simulink model "robot_etu"  (R2022a)
settings: Solver=VariableStepAuto  StartTime=0.0  StopTime=10  RelTol=1e-3
values from neighbouring files (symbols this model uses):
  K = -place(A,B,V)    [matrices.m]
undefined symbols (not defined in the file or in its folder): DiscIntNeverNeededParam, ue, x0, xe
libraries: simulink x1
settings Model: Creator=acanon  LastModifiedBy=acanon

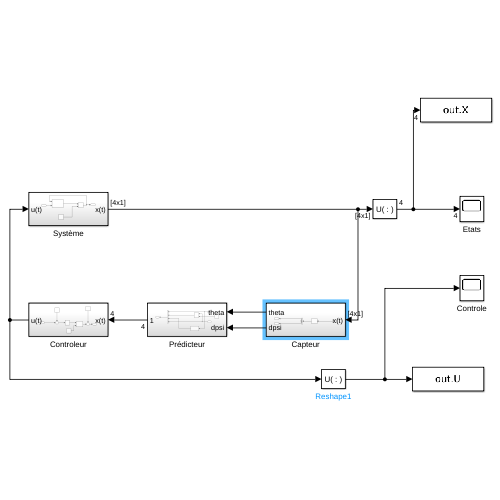
[thumbnail: Simulink's stored preview of the top-level diagram]
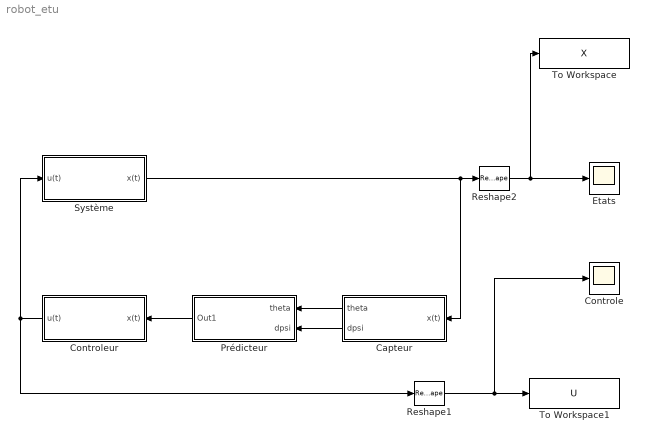
== system robot_etu ==
  Capteur : Subsystem
  Controle : Scope
  Controleur : Subsystem
  Etats : Scope
  Prédicteur : Subsystem
  Reshape1 : Reshape
  Reshape2 : Reshape
  Système : Subsystem
  To Workspace : ToWorkspace  VariableName=X  SaveFormat=Timeseries  SampleTime=-1
  To Workspace1 : ToWorkspace  VariableName=U  SaveFormat=Timeseries  SampleTime=-1
  wires:
  Controleur/1(u(t)) -> Système/1(u(t)), Reshape1/1
  Prédicteur/1(Out1) -> Controleur/1(x(t))
  Capteur/1(theta) -> Prédicteur/1(theta)
  Capteur/2(dpsi) -> Prédicteur/2(dpsi)
  Système/1(x(t)) -> Capteur/1(x(t)), Reshape2/1
  Reshape2/1 -> To Workspace/1, Etats/1
  Reshape1/1 -> Controle/1, To Workspace1/1

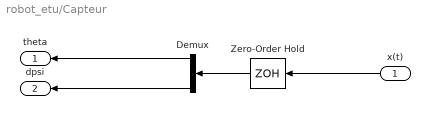
== system robot_etu/Capteur ==
  x(t) : Inport
  Demux : Demux
  Zero-Order Hold : ZeroOrderHold  SampleTime=-1
  theta : Outport
  dpsi : Outport  Port=2
  wires:
  x(t)/1 -> Zero-Order Hold/1
  Demux/1 -> theta/1
  Demux/4 -> dpsi/1
  Zero-Order Hold/1 -> Demux/1

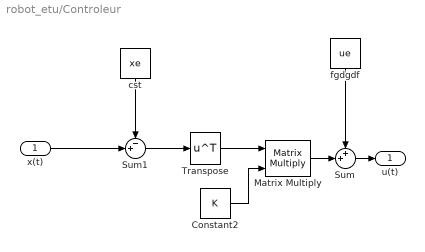
== system robot_etu/Controleur ==
  x(t) : Inport
  Constant2 : Constant  Value=K
  Matrix Multiply : Product  Multiplication=Matrix(*)
  Sum : Sum  Inputs=++|
  Sum1 : Sum  Inputs=-+|
  Transpose : Math  Operator=transpose
  cst : Constant  Value=xe
  fgdgdf : Constant  Value=ue
  u(t) : Outport
  wires:
  fgdgdf/1 -> Sum/1
  x(t)/1 -> Sum1/2
  Sum/1 -> u(t)/1
  Matrix Multiply/1 -> Sum/2
  cst/1 -> Sum1/1
  Constant2/1 -> Matrix Multiply/2
  Sum1/1 -> Transpose/1
  Transpose/1 -> Matrix Multiply/1

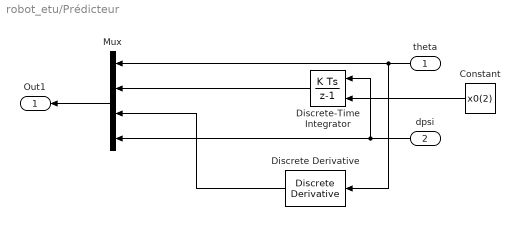
== system robot_etu/Prédicteur ==
  theta : Inport
  dpsi : Inport  Port=2
  Constant : Constant  Value=x0(2)
  Discrete Derivative : simulink/Discrete/Discrete Derivative  gainval=1.0  ICPrevScaledInput=0.0  OutMin=[]  OutMax=[]  OutDataType=fixdt(1, 16)  OutScaling=2^-10  DoSatur=off
  Discrete-Time Integrator : DiscreteIntegrator  InitialConditionSource=external  SampleTime=-1  ICPrevOutput=DiscIntNeverNeededParam  ICPrevScaledInput=DiscIntNeverNeededParam
  Mux : Mux
  Out1 : Outport
  wires:
  theta/1 -> Discrete Derivative/1, Mux/1
  dpsi/1 -> Discrete-Time Integrator/1, Mux/4
  Constant/1 -> Discrete-Time Integrator/2
  Discrete-Time Integrator/1 -> Mux/2
  Discrete Derivative/1 -> Mux/3
  Mux/1 -> Out1/1

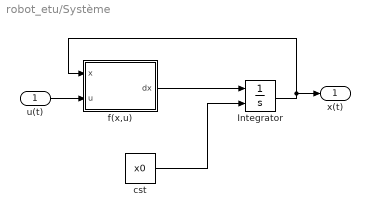
== system robot_etu/Système ==
  u(t) : Inport
  Integrator : Integrator  InitialConditionSource=external
  cst : Constant  Value=x0
  f(x,u) : MATLAB Function  TreatAsAtomicUnit=on
  x(t) : Outport
  wires:
  u(t)/1 -> f(x,u)/2(u)
  f(x,u)/1(dx) -> Integrator/1
  Integrator/1 -> f(x,u)/1(x), x(t)/1
  cst/1 -> Integrator/2

== matlab function robot_etu/Système/f(x,u) ==
  data: x input; u input; dx output
function dx   = fonction( x, u)
%   Dynamic equations of motion of the segway on an axis.
%   Inputs: - x = [theta psi dtheta dpsi]
%               theta: average angle of the wheels      [rad]
%               psi: body pitch angle                   [rad]
%               dtheta: average velocity of the wheels  [rad/s]
%               dpsi: body pitch velocity               [rad/s]
%          - u: DC motor voltage (same value for both motors) [V]

    % State
    psi = x(2);
    dtheta = x(3);
    dpsi = x(4);

    % Parameters
    
    g = 9.81;           % gravity acceleration [m/sec^2]
    m = 0.03;           % wheel weight [kg]
    R = 0.04;           % wheel radius [m]
    Jw = m*R^2/2;       % wheel inertia moment [kg*m^2]
    M = 0.6;            % body weight [kg]
    H = 0.144;          % body height [m]
    L = H/2;            % distance of the center of mass from the wheel axle [m]
    Jpsi = M*L^2/3;     % body pitch inertia [kgm^2]
    Jm = 1e-5;          % DC motor inertia moment [kgm^2]
    Rm = 6.69;          % DC motor resistance [Ohm]
    Kb = 0.468;         % DC motor back EMF constant [Vsec/rad]
    Kt = 0.317;         % DC motor torque constant [Nm/A]
    n = 1;              % gear ratio
    fm = 0.0022;        % friction coefficient between body and DC motor
    fw = 0;             % friction coefficient between wheel and floor
    
    % Equations of motion
    c1 = (2*m+M)*R^2 + 2*Jw + 2*n^2*Jm;
    c2 = M*L*R*cos(psi) - 2*n^2*Jm;
    c3 = -M*L*R*dpsi^2*sin(psi);
    c4 = M*L^2 + Jpsi + 2*n^2*Jm;
    c5 = -M*g*L*sin(psi);

    alpha = Kt/Rm;
    beta = Kt*Kb/Rm + fm;

    Ftheta = alpha*(2*u) - 2*(beta+fw)*dtheta + 2*beta*dpsi;
    Fpsi = -alpha*(2*u) + 2*beta*dtheta - 2*beta*dpsi;

    ddtheta = (c4*c3 - c2*c5 + c4*Ftheta - c2*Fpsi)/(c4*c1 - c2^2);
    ddpsi = (Fpsi- c2*ddtheta - c5)/c4;
    dx = [dtheta dpsi ddtheta ddpsi]';

end
